simulink model "dpace_test"  (Simulink 4.00)
settings: Solver=FixedStepDiscrete  StartTime=0.0  StopTime=inf  FixedStep=0.001  RelTol=1e-3
PostLoadFcn:
  | ,try, rti_mdl_postloadfcn(bdroot, 'UpdateModel', 25, 'RTI1102'); catch, disp(lasterr); end,
libraries: rtilib1102 x2
settings Model: LastModifiedBy=fodor  SimulationMode=external  RTWSystemTargetFile=rti1102.tlc  RTWRetainRTWFile=on  RTWTemplateMakefile=rti1102.tmf  RTWMakeCommand=make_rti  ExtModeMexFile=rti_comm  OptimizeBlockIOStorage=off  BlockReductionOpt=off

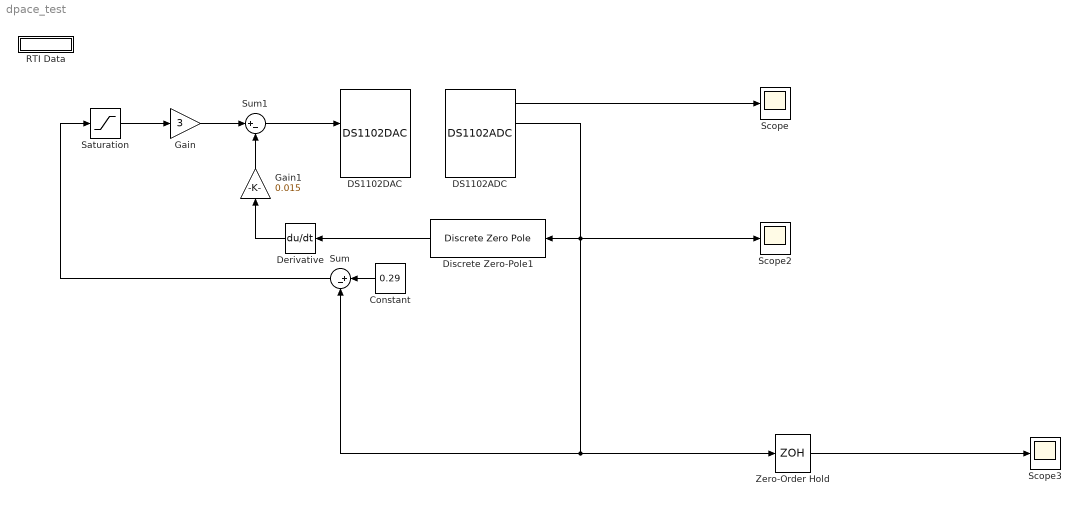
== system dpace_test ==
  Constant : Constant  Orientation=left  Value=0.29
  DS1102ADC : rtilib1102/DS1102/DS1102ADC  DialogFcn=gui1102adc  UnitName={ 'DS1102ADC' }  UnitValues={ [] }  DSProperties=struct('RTI',struct('Version',uint32(1),'BlockType',struct('isSLSource',uint8(1),'isSLSink',uint8(0),'isHWSource',uint8(1),'isHWSink',uint8(0),'isSetup',uint8(0),'isInline',uint8(1),'isNonInline',uint8(0),'isInterrupt',uint8(0),'isChannelwise',uint8(0)),'IOBoardType','DS1102','UnitType','ADC','Identifier','ADC','DialogType','ML','BlockSet','NONE','SlaveProcessor','NONE'))
  DS1102DAC : rtilib1102/DS1102/DS1102DAC  Range=[10 10 10 10]  InitValue=[0 0 0 0]  TermMode=[1 1 1 1]  TermValue=[0 0 0 0]  DialogFcn=gui1102dac  UnitName={ 'DS1102DAC' }  UnitValues={ [] }  DSProperties=struct('RTI',struct('Version',uint32(1),'BlockType',struct('isSLSource',uint8(0),'isSLSink',uint8(1),'isHWSource',uint8(0),'isHWSink',uint8(1),'isSetup',uint8(0),'isInline',uint8(1),'isNonInline',uint8(0),'isInterrupt',uint8(0),'isChannelwise',uint8(0)),'IOBoardType','DS1102','UnitType','DAC','Identifier','DAC','DialogType','ML','BlockSet','NONE','SlaveProcessor','NONE'))
  Derivative : Derivative  Orientation=left
  Discrete Zero-Pole1 : DiscreteZeroPole  Orientation=left  Zeros=[-1 -1]  Poles=[0.9555985337+1i*0.0425120826 0.9555985337-1i*0.0425120826]  Gain=1/1.058546241e+03  SampleTime=0.001
  Gain : Gain  Gain=3  Multiplication=Element-wise(K.*u)  SaturateOnIntegerOverflow=on
  Gain1 : Gain  Orientation=up  Gain=0.015  Multiplication=Element-wise(K.*u)  SaturateOnIntegerOverflow=on
  RTI Data : Subsystem  Tag=struct('RTIDataServer',struct('RTIDataServerVs','2','RTIModelDescription','struct(''main'',''dpace_test'',''sub'','''',''isMp'',0)'))  LoadFcn="try,  rtidc('DataHostBlockClbLoad', gcbh); catch, disp(['Warning: ''LoadFcn'' for RTI Data block failed: ' lasterr]); end"
      settings: CopyFcn="try,  rtidc('DataHostBlockClbCopy', gcbh); catch, disp(['Warning: ''CopyFcn'' for RTI Data block failed: ' lasterr]); end"  DeleteFcn="try,  rtidc('DataHostBlockClbDelete', gcbh); catch, disp(['Warning: ''DeleteFcn'' for RTI Data block failed: ' lasterr]); end"  ModelCloseFcn="try,  rtidc('DataHostBlockClbModelClose', gcbh); catch, disp(['Warning: ''ModelCloseFcn'' for RTI Data block failed: ' lasterr]); end"  PreSaveFcn="try,  rtidc('DataHostBlockClbPreSave', gcbh); catch, disp(['Warning: ''PreSaveFcn'' for RTI Data block failed: ' lasterr]); end"  PostSaveFcn="try,  rtidc('DataHostBlockClbPostSave', gcbh); catch, disp(['Warning: ''PostSaveFcn'' for RTI Data block failed: ' lasterr]); end"  NameChangeFcn="try,  rtidc('DataHostBlockClbNameChange', gcbh); catch, disp(['Warning: ''NameChangeFcn'' for RTI Data block failed: ' lasterr]); end"  RTWFcnNameOpts=Auto  RTWFileNameOpts=Auto
      mask Type: RTI_DATA_HOST
      mask Description:
      | RTI Data Block.
      | This block is used by RTI to store internal model-dependent data.
      | Please keep this block on the root level of the model. Deleting this block will result in data loss.
      | 
      | NEVER DELETE OR COPY THIS BLOCK!
      mask Help:
      | RTI Data Block.
      | This block is used by RTI to store internal model-dependent data.
      | Please keep this block on the root level of the model. Deleting this block will result in data loss.
      | 
      | NEVER DELETE OR COPY THIS BLOCK!
      mask Display: text(0.5, 0.5, 'RTI Data', 'HorizontalAlignment', 'center');
  Saturation : Saturate  UpperLimit=0.1  LowerLimit=0  LinearizeAsGain=on
  Scope : Scope
      settings: TimeRange=auto  YMin=-1  YMax=1  SaveToWorkspace=off  SaveName=ScopeData  LimitDataPoints=on  MaxDataPoints=5000
  Scope2 : Scope
      settings: TimeRange=auto  YMin=-1  YMax=1  SaveToWorkspace=off  SaveName=ScopeData2  LimitDataPoints=on  MaxDataPoints=5000  SampleInput=on  SampleTime=0.001
  Scope3 : Scope
      settings: TimeRange=auto  YMin=-1  YMax=1  SaveToWorkspace=off  SaveName=ScopeData3  LimitDataPoints=on  MaxDataPoints=5000  SampleInput=on  SampleTime=1/10
  Sum : Sum  Orientation=left  Inputs=|+-  SaturateOnIntegerOverflow=on
  Sum1 : Sum  Inputs=|+-  SaturateOnIntegerOverflow=on
  Zero-Order Hold : ZeroOrderHold  SampleTime=1/10
  wires:
  DS1102ADC/1 -> Scope/1
  Sum/1 -> Saturation/1
  Constant/1 -> Sum/1
  Saturation/1 -> Gain/1
  DS1102ADC/2 -> Discrete Zero-Pole1/1, Scope2/1, Sum/2, Zero-Order Hold/1
  Discrete Zero-Pole1/1 -> Derivative/1
  Gain/1 -> Sum1/1
  Sum1/1 -> DS1102DAC/2
  Derivative/1 -> Gain1/1
  Gain1/1 -> Sum1/2
  Zero-Order Hold/1 -> Scope3/1

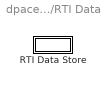
== system dpace_test/RTI Data ==
  RTI Data Store : Subsystem  Tag="struct('private',struct('version',struct('dsVer',uint32(2),'dsVerCreation',uint32(2),'RTI',struct('ver','4.1','type','RTI1102')),'access',struct('type','Model','isPerm',1,'created',['12-Sep-2011 13:51:55'],'modified',['14-Dec-2011 16:18:14'],'location','')),'public',struct('main',struct('data',[]),'sub',struct('name',{{'dpace_test'}},'data',{{struct('TH',struct('thTaskInfo',struct('taskType',{'TIMER','HWINT','TMRINT','SWINT'},'tasksNumOf',{2,0,0,0},'srcIds',{{'TIMERA','TIMERA2'},{},{},{}},'taskNames',{{['Timer Task 1'],['Timer Task 2']},{},{},{}})),'th_tc',struct('taskType',{'TIMER','TIMER'},'blkh',{-1,-1},'srcId',{'TIMERA','TIMERA2'},'srcSgnName',{['Timer A interrupt'],['Timer Task 1']},'srcCpuName',{'',''},'taskName',{['Timer Task 1  [0.001] s'],['Timer Task 2  [0.1] s']},'smplTime',{1e-03,1.0000000000000001e-01},'smplTimeOffs',{0,0},'priority',{1,2},'ovcType',{1,1},'ovcMax',{0,0}),'tc_th',struct('taskType',{'TIMER','TIMER'},'blkh',{-1,-1},'srcId',{'TIMERA','TIMERA2'},'srcSgnName',{['Timer A interrupt'],['Timer Task 1']},'srcCpuName',{'',''},'taskName',{['Timer Task 1  [0.001] s'],['Timer Task 2  [0.1] s']},'smplTime',{1e-03,1.0000000000000001e-01},'smplTimeOffs',{0,0},'priority',{1,2},'ovcType',{1,1},'ovcMax',{0,0}))}})))"
      settings: RTWFcnNameOpts=Auto  RTWFileNameOpts=Auto
      mask Type: RTI_DATA_STORE
      mask Description:
      | RTI Data Store Block. This block is used by RTI to store internal model dependent data. Deleting this block will result in data loss.
      | 
      | NEVER DELETE, COPY, OR MODIFY THIS BLOCK!
      mask Help:
      | RTI Data Store Block. This block is used by RTI to store internal model dependent data. Deleting this block will result in data loss.
      | 
      | NEVER DELETE, COPY, OR MODIFY THIS BLOCK!
      mask Display: text(0.5, 0.5, ' ', 'HorizontalAlignment', 'center');

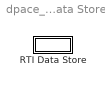
== system dpace_test/RTI Data/RTI Data Store ==
  RTI Data Store : Subsystem
      settings: RTWFcnNameOpts=Auto  RTWFileNameOpts=Auto
      mask Type: RTI_DATA_STORE
      mask Description:
      | RTI Data Store Block. This block is used by RTI to store internal model dependent data. Deleting this block will result in data loss.
      | 
      | NEVER DELETE, COPY, OR MODIFY THIS BLOCK!
      mask Help:
      | RTI Data Store Block. This block is used by RTI to store internal model dependent data. Deleting this block will result in data loss.
      | 
      | NEVER DELETE, COPY, OR MODIFY THIS BLOCK!
      mask Display: text(0.5, 0.5, ' ', 'HorizontalAlignment', 'center');

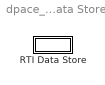
== system dpace_test/RTI Data/RTI Data Store/RTI Data Store ==
  RTI Data Store : Subsystem
      settings: RTWFcnNameOpts=Auto  RTWFileNameOpts=Auto
      mask Type: RTI_DATA_STORE
      mask Description:
      | RTI Data Store Block. This block is used by RTI to store internal model dependent data. Deleting this block will result in data loss.
      | 
      | NEVER DELETE, COPY, OR MODIFY THIS BLOCK!
      mask Help:
      | RTI Data Store Block. This block is used by RTI to store internal model dependent data. Deleting this block will result in data loss.
      | 
      | NEVER DELETE, COPY, OR MODIFY THIS BLOCK!
      mask Display: text(0.5, 0.5, ' ', 'HorizontalAlignment', 'center');

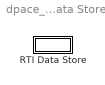
== system dpace_test/RTI Data/RTI Data Store/RTI Data Store/RTI Data Store ==
  RTI Data Store : Subsystem
      settings: RTWFcnNameOpts=Auto  RTWFileNameOpts=Auto
      mask Type: RTI_DATA_STORE
      mask Description:
      | RTI Data Store Block. This block is used by RTI to store internal model dependent data. Deleting this block will result in data loss.
      | 
      | NEVER DELETE, COPY, OR MODIFY THIS BLOCK!
      mask Help:
      | RTI Data Store Block. This block is used by RTI to store internal model dependent data. Deleting this block will result in data loss.
      | 
      | NEVER DELETE, COPY, OR MODIFY THIS BLOCK!
      mask Display: text(0.5, 0.5, ' ', 'HorizontalAlignment', 'center');

== system dpace_test/RTI Data/RTI Data Store/RTI Data Store/RTI Data Store/RTI Data Store ==
